simulink model "filterbankFIR"  (R2018a)
settings: Solver=FixedStepDiscrete  StartTime=0.0  StopTime=0.01  RelTol=1e-3
values from neighbouring files (symbols this model uses):
  gainConsts = 10.^(requiredGainDB/10)    [main.m]
  T = table(Band, fm, Lowerfreq, Upperfreq, Fstop2, Fstop1)    [filterbankProto.m]    (also in main.m = 2.26757369615e-05)
undefined symbols (not defined in the file or in its folder): fdesignblkfcn, gcbh
libraries: dspsrcs4 x2, dspfdesign x2, dspxfrm3 x1, dspspect3 x1, dspsigops x1, dspmisc x1, dspmtrx3 x1, dspobslib x1
(part 1 of 5)
settings Model: SimulationMode=accelerator  Creator=Kavi  LastModifiedBy=kavilannair
settings SolverCC: AutoInsertRateTranBlk=on
settings DataIOCC: LimitDataPoints=on  SaveOutput=off  SignalLogging=off  SaveTime=off
settings OptimizationCC: LifeSpan=inf  SimCompilerOptimization=on
settings DebuggingCC: AlgebraicLoopMsg=error  SingleTaskRateTransMsg=error  AllowSymbolicDim=off  SFUnexpectedBacktrackingDiag=warning  SFNoUnconditionalDefaultTransitionDiag=warning  SFExecutionAtInitializationDiag=none
settings CodeAppCC: StateflowObjectComments=on
settings GRTTargetCC: TargetLangStandard=C89/C90 (ANSI)  GeneratePreprocessorConditionals=Disable all
settings ConfigComp: CovMetricSettings=dw  CovHtmlReporting=on  CovSaveCumulativeToWorkspaceVar=on  CovSaveSingleToWorkspaceVar=on  CovExternalEMLEnable=off  CovSFcnEnable=off

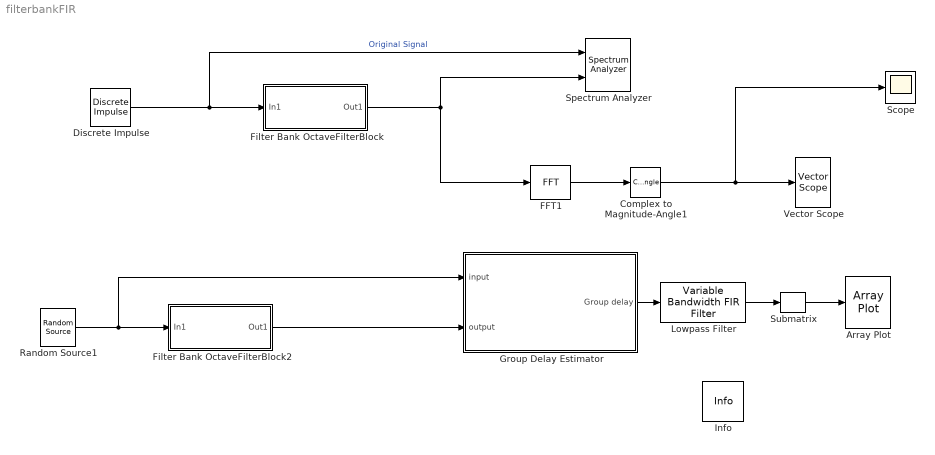
== system filterbankFIR ==
  Array Plot : ArrayPlot
  Complex to Magnitude-Angle1 : ComplexToMagnitudeAngle  Output=Magnitude
  Discrete Impulse : dspsrcs4/Discrete  Impulse  Delay=0  SampleTime=T  FrameSample=512  OutputFrames=off  dataType=double  isSigned=on  wordLen=16  udDataType=sfix(16)  fracBitsMode=Best precision  numFracBits=15  OutDataTypeStr=double  LastOutDataTypeStr=double
  FFT1 : dspxfrm3/FFT  FFTImplementation=Auto  CompMethod=Table lookup  TableOpt=NEW  TableOptActive=Speed  BitRevOrder=off  Normalize=off  InheritFFTLength=on  FFTLength=64  WrapInput=on  roundingMode=Floor  overflowMode=off  firstCoeffDataTypeStr=Inherit: Same word length as input  firstCoeffLastDataTypeStr=Inherit: Same word length as input  outputMin=[]  outputMax=[]
  Filter Bank OctaveFilterBlock : Subsystem
  Filter Bank OctaveFilterBlock2 : Subsystem
  Group Delay Estimator : Subsystem
  Info : dspmisc/Info  SystemSampleTime=-1
      settings: SourceProductName=DSP System Toolbox  SourceProductBaseCode=DS
  Lowpass Filter : dspfdesign/Variable Bandwidth FIR Filter  FilterOrder=30  FilterType=Lowpass  CutoffFrequencyPort=off  CutoffFrequency=fc  CenterFrequencyPort=off  CenterFrequency=1e4  BandwidthPort=off  Bandwidth=2e3  Window=Hann  KaiserWindowParameter=.5  SidelobeAttenuation=60  InheritSampleRate=off  SampleRate=44100  SimulateUsing=Interpreted execution  mask(dsp.simulink.VariableBandwidthFIRFilter){fc=1323.094}
      mask prompts: fc "Cutoff frequency (Hz)"
      mask help: Masked version of dspfdesign/Variable Bandwidth FIR Filter block
      settings: SourceProductName=DSP System Toolbox  SourceProductBaseCode=DS
      mask Display:
      | % This is a new mask on top of the base mask.
      | % Use "View base mask" link below to see the base mask.
      | fprintf('Lowpass filter')
  Random Source1 : dspsrcs4/Random Source  SrcType=Gaussian  NormMethod=Ziggurat  CltLength=12  MinVal=0  MaxVal=1  MeanVal=0  VarVal=1  RepMode=Repeatable  rawSeed=1  IsInherit=off  SampMode=Discrete  SampTime=1/44100  SampFrame=512  DataType=Double  OutComplex=Real  OutputFrames=off
  Scope : Scope
  Spectrum Analyzer : SpectrumAnalyzer  NumInputPorts=2
  Submatrix : dspmtrx3/Submatrix  RowSpan=Range of rows  RowStartMode=Index  RowStartIndex=31  RowEndMode=Last  RowEndIndex=1  ColSpan=All columns  ColStartMode=First  ColStartIndex=1  ColEndMode=Last  ColEndIndex=1
  Vector Scope : dspobslib/Vector Scope  ScopeProperties=off  Domain=Frequency  HorizSpan=1  DisplayProperties=off  AxisGrid=on  Memory=off  FrameNumber=on  AxisLegend=off  AxisZoom=off  OpenScopeAtSimStart=on  OpenScopeImmediately=off  FigPos=[86 244 1118 420]  AxisProperties=on  XUnits=Hertz  XRange=[0...Fs/2]  InheritXIncr=on  XIncr=1  XLabel=Samples  XLimit=Auto  XMin=0  XMax=1  XStart=0  YUnits=dB  YLabel=|Magnitude (dB)|  LineProperties=off  LineMarkers=+  LineColors=[1 0 0]  XAxisParamsVer=6.9
      settings: SourceProductName=DSP System Toolbox  SourceProductBaseCode=DS  YMin=0.0723692553519949  YMax=69.3188381671759
  wires:
  Discrete Impulse/1 -> Spectrum Analyzer/1, Filter Bank OctaveFilterBlock/1(In1)  "Original Signal"
  Complex to Magnitude-Angle1/1 -> Scope/1, Vector Scope/1
  FFT1/1 -> Complex to Magnitude-Angle1/1
  Filter Bank OctaveFilterBlock/1(Out1) -> FFT1/1, Spectrum Analyzer/2
  Filter Bank OctaveFilterBlock2/1(Out1) -> Group Delay Estimator/2(output)
  Group Delay Estimator/1(Group delay) -> Lowpass Filter/1
  Submatrix/1 -> Array Plot/1
  Lowpass Filter/1 -> Submatrix/1
  Random Source1/1 -> Filter Bank OctaveFilterBlock2/1(In1), Group Delay Estimator/1(input)

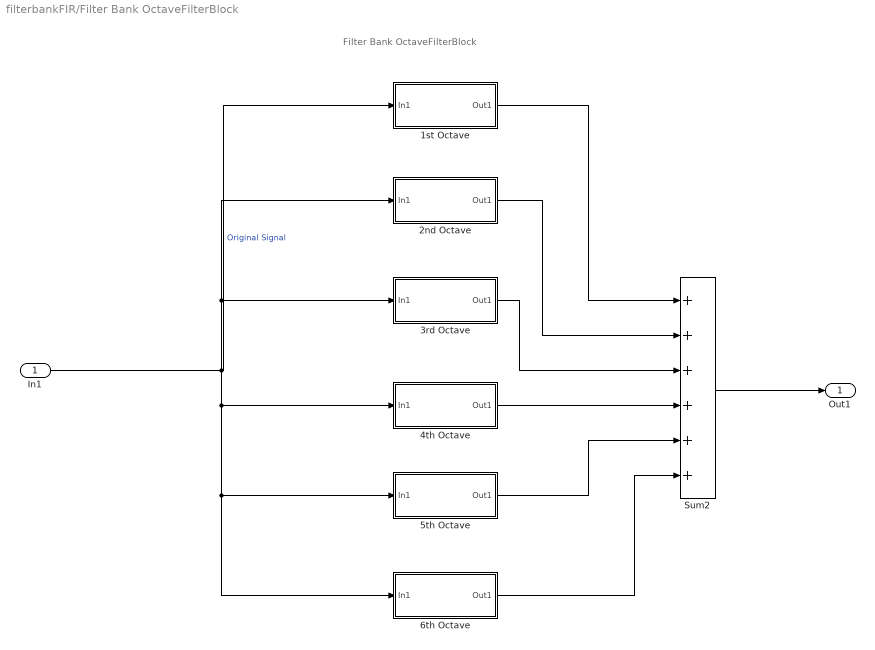
== system filterbankFIR/Filter Bank OctaveFilterBlock ==
  note: Filter Bank OctaveFilterBlock
  In1 : Inport
  "1st Octave " : Subsystem
  2nd Octave : Subsystem
  "3rd Octave " : Subsystem
  4th Octave : Subsystem
  5th Octave : Subsystem
  6th Octave : Subsystem
  Sum2 : Sum  Inputs=++++++
  Out1 : Outport
  wires:
  Sum2/1 -> Out1/1
  "1st Octave "/1(Out1) -> Sum2/1
  2nd Octave/1(Out1) -> Sum2/2
  "3rd Octave "/1(Out1) -> Sum2/3
  4th Octave/1(Out1) -> Sum2/4
  5th Octave/1(Out1) -> Sum2/5
  6th Octave/1(Out1) -> Sum2/6
  In1/1 -> 4th Octave/1(In1), 5th Octave/1(In1), 6th Octave/1(In1), "3rd Octave "/1(In1), 2nd Octave/1(In1), "1st Octave "/1(In1)  "Original Signal"

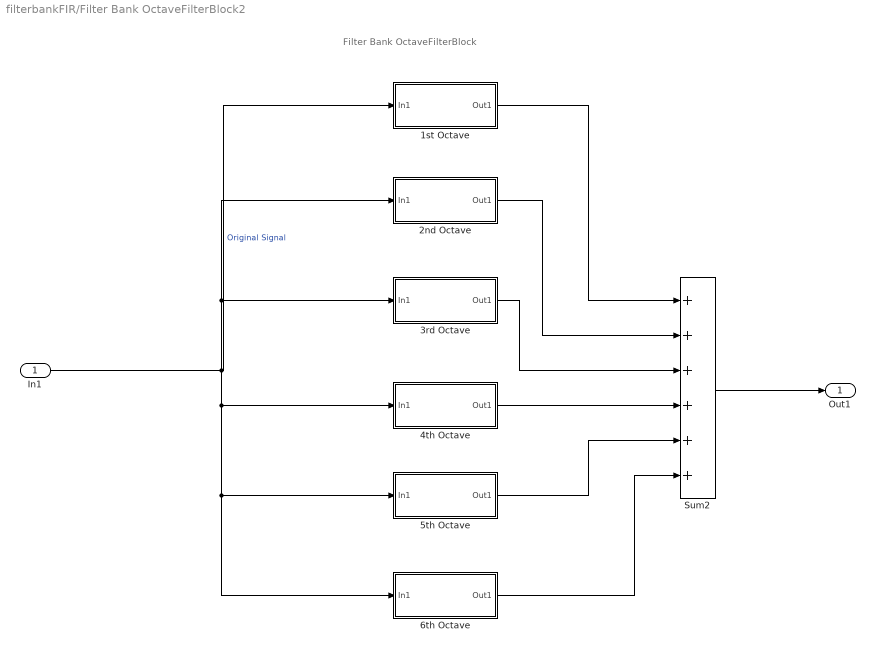
== system filterbankFIR/Filter Bank OctaveFilterBlock2 ==
  note: Filter Bank OctaveFilterBlock
  In1 : Inport
  "1st Octave " : Subsystem
  2nd Octave : Subsystem
  "3rd Octave " : Subsystem
  4th Octave : Subsystem
  5th Octave : Subsystem
  6th Octave : Subsystem
  Sum2 : Sum  Inputs=++++++
  Out1 : Outport
  wires:
  Sum2/1 -> Out1/1
  "1st Octave "/1(Out1) -> Sum2/1
  2nd Octave/1(Out1) -> Sum2/2
  "3rd Octave "/1(Out1) -> Sum2/3
  4th Octave/1(Out1) -> Sum2/4
  5th Octave/1(Out1) -> Sum2/5
  6th Octave/1(Out1) -> Sum2/6
  In1/1 -> 4th Octave/1(In1), 5th Octave/1(In1), 6th Octave/1(In1), "3rd Octave "/1(In1), 2nd Octave/1(In1), "1st Octave "/1(In1)  "Original Signal"

== system filterbankFIR/Group Delay Estimator ==
  input : Inport
  output : Inport  Port=2
  Differentiator Filter : dspfdesign/Differentiator Filter  DesignForMinimumOrder=off  FilterOrder=3  PassbandRipple=0.1  ScaleCoefficients=off  SimulateUsing=Interpreted execution  roundingMode=Floor  coeffsDataTypeStr=fixdt(1,16)
      settings: SourceProductName=DSP System Toolbox  SourceProductBaseCode=DS
  Discrete Transfer Function Estimator : dspspect3/Discrete Transfer Function Estimator  WindowLength=2056  Overlap=0  SpectralAverages=10  FFTLengthSource=Auto  FFTLength=2048  Window=Hann  SidelobeAttenuation=60  FrequencyRange=One-sided  OutputCoherence=off  SimulateUsing=Code generation
      settings: SourceProductName=DSP System Toolbox  SourceProductBaseCode=DS
  Gain1 : Gain  Gain=-22050/257
  Phase Extractor : dspsigops/Phase Extractor  TreatFramesIndependently=on  SimulateUsing=Code generation
      settings: SourceProductName=DSP System Toolbox  SourceProductBaseCode=DS
  Group delay : Outport
  wires:
  output/1 -> Discrete Transfer Function Estimator/2
  Differentiator Filter/1 -> Group delay/1
  input/1 -> Discrete Transfer Function Estimator/1
  Gain1/1 -> Differentiator Filter/1
  Phase Extractor/1 -> Gain1/1
  Discrete Transfer Function Estimator/1 -> Phase Extractor/1

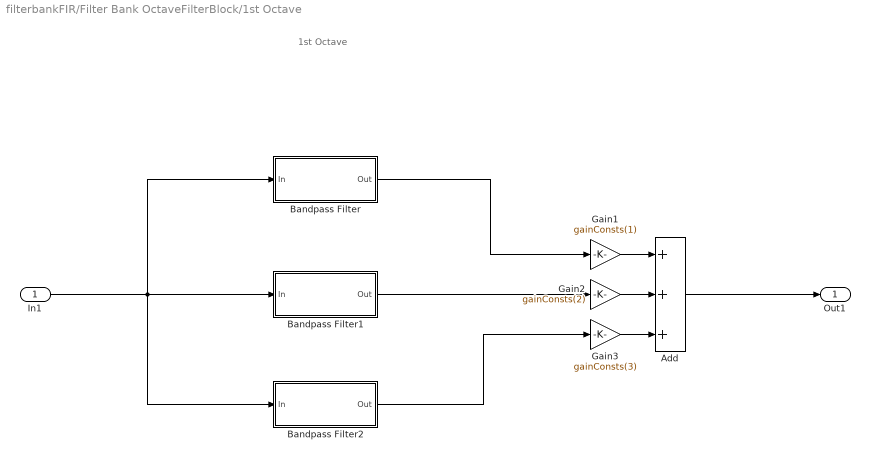
== system filterbankFIR/Filter Bank OctaveFilterBlock/1st Octave  ==
  note: 1st Octave
  In1 : Inport
  Add : Sum  Inputs=+++
  Bandpass Filter : Subsystem  DialogController=fdesignblkfcn  InitFcn=fdesignblkfcn(gcbh, {'InitFcn'});  mask(Bandpass Filter){}
      mask help: Design a bandpass filter
      settings: CopyFcn=fdesignblkfcn(gcbh, {'CopyFcn'});
      mask Help: helpview(mapfilelocation('dsp'), 'dspbandpassfilter');
      mask Display: disp('Bandpass');
  Bandpass Filter1 : Subsystem  DialogController=fdesignblkfcn  InitFcn=fdesignblkfcn(gcbh, {'InitFcn'});  mask(Bandpass Filter){}
      mask help: Design a bandpass filter
      settings: CopyFcn=fdesignblkfcn(gcbh, {'CopyFcn'});
      mask Help: helpview(mapfilelocation('dsp'), 'dspbandpassfilter');
      mask Display: disp('Bandpass');
  Bandpass Filter2 : Subsystem  DialogController=fdesignblkfcn  InitFcn=fdesignblkfcn(gcbh, {'InitFcn'});  mask(Bandpass Filter){}
      mask help: Design a bandpass filter
      settings: CopyFcn=fdesignblkfcn(gcbh, {'CopyFcn'});
      mask Help: helpview(mapfilelocation('dsp'), 'dspbandpassfilter');
      mask Display: disp('Bandpass');
  Gain1 : Gain  Gain=gainConsts(1)
  Gain2 : Gain  Gain=gainConsts(2)
  Gain3 : Gain  Gain=gainConsts(3)
  Out1 : Outport
  wires:
  In1/1 -> Bandpass Filter2/1(In), Bandpass Filter1/1(In), Bandpass Filter/1(In)
  Bandpass Filter1/1(Out) -> Gain2/1
  Bandpass Filter/1(Out) -> Gain1/1
  Bandpass Filter2/1(Out) -> Gain3/1
  Add/1 -> Out1/1
  Gain1/1 -> Add/1
  Gain2/1 -> Add/2
  Gain3/1 -> Add/3

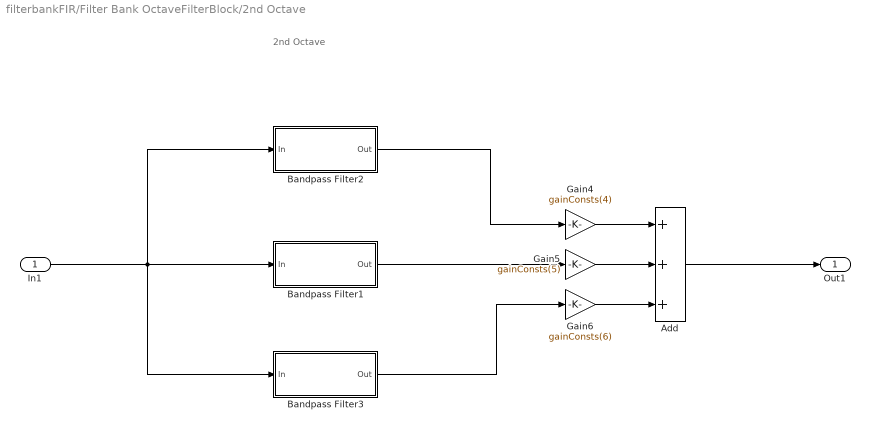
== system filterbankFIR/Filter Bank OctaveFilterBlock/2nd Octave ==
  note: 2nd Octave
  In1 : Inport
  Add : Sum  Inputs=+++
  Bandpass Filter1 : Subsystem  DialogController=fdesignblkfcn  InitFcn=fdesignblkfcn(gcbh, {'InitFcn'});  mask(Bandpass Filter){}
      mask help: Design a bandpass filter
      settings: CopyFcn=fdesignblkfcn(gcbh, {'CopyFcn'});
      mask Help: helpview(mapfilelocation('dsp'), 'dspbandpassfilter');
      mask Display: disp('Bandpass');
  Bandpass Filter2 : Subsystem  DialogController=fdesignblkfcn  InitFcn=fdesignblkfcn(gcbh, {'InitFcn'});  mask(Bandpass Filter){}
      mask help: Design a bandpass filter
      settings: CopyFcn=fdesignblkfcn(gcbh, {'CopyFcn'});
      mask Help: helpview(mapfilelocation('dsp'), 'dspbandpassfilter');
      mask Display: disp('Bandpass');
  Bandpass Filter3 : Subsystem  DialogController=fdesignblkfcn  InitFcn=fdesignblkfcn(gcbh, {'InitFcn'});  mask(Bandpass Filter){}
      mask help: Design a bandpass filter
      settings: CopyFcn=fdesignblkfcn(gcbh, {'CopyFcn'});
      mask Help: helpview(mapfilelocation('dsp'), 'dspbandpassfilter');
      mask Display: disp('Bandpass');
  Gain4 : Gain  Gain=gainConsts(4)
  Gain5 : Gain  Gain=gainConsts(5)
  Gain6 : Gain  Gain=gainConsts(6)
  Out1 : Outport
  wires:
  In1/1 -> Bandpass Filter3/1(In), Bandpass Filter1/1(In), Bandpass Filter2/1(In)
  Bandpass Filter1/1(Out) -> Gain5/1
  Bandpass Filter2/1(Out) -> Gain4/1
  Bandpass Filter3/1(Out) -> Gain6/1
  Add/1 -> Out1/1
  Gain4/1 -> Add/1
  Gain5/1 -> Add/2
  Gain6/1 -> Add/3

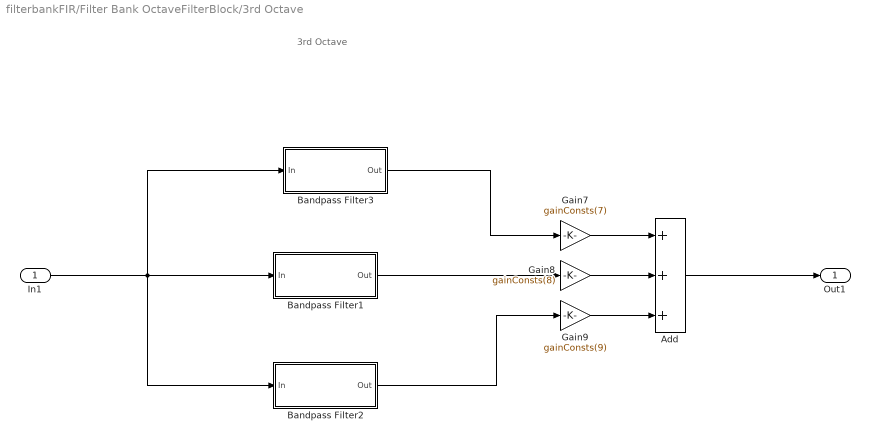
== system filterbankFIR/Filter Bank OctaveFilterBlock/3rd Octave  ==
  note: 3rd Octave
  In1 : Inport
  Add : Sum  Inputs=+++
  Bandpass Filter1 : Subsystem  DialogController=fdesignblkfcn  InitFcn=fdesignblkfcn(gcbh, {'InitFcn'});  mask(Bandpass Filter){}
      mask help: Design a bandpass filter
      settings: CopyFcn=fdesignblkfcn(gcbh, {'CopyFcn'});
      mask Help: helpview(mapfilelocation('dsp'), 'dspbandpassfilter');
      mask Display: disp('Bandpass');
  Bandpass Filter2 : Subsystem  DialogController=fdesignblkfcn  InitFcn=fdesignblkfcn(gcbh, {'InitFcn'});  mask(Bandpass Filter){}
      mask help: Design a bandpass filter
      settings: CopyFcn=fdesignblkfcn(gcbh, {'CopyFcn'});
      mask Help: helpview(mapfilelocation('dsp'), 'dspbandpassfilter');
      mask Display: disp('Bandpass');
  Bandpass Filter3 : Subsystem  DialogController=fdesignblkfcn  InitFcn=fdesignblkfcn(gcbh, {'InitFcn'});  mask(Bandpass Filter){}
      mask help: Design a bandpass filter
      settings: CopyFcn=fdesignblkfcn(gcbh, {'CopyFcn'});
      mask Help: helpview(mapfilelocation('dsp'), 'dspbandpassfilter');
      mask Display: disp('Bandpass');
  Gain7 : Gain  Gain=gainConsts(7)
  Gain8 : Gain  Gain=gainConsts(8)
  Gain9 : Gain  Gain=gainConsts(9)
  Out1 : Outport
  wires:
  In1/1 -> Bandpass Filter2/1(In), Bandpass Filter1/1(In), Bandpass Filter3/1(In)
  Bandpass Filter1/1(Out) -> Gain8/1
  Bandpass Filter3/1(Out) -> Gain7/1
  Bandpass Filter2/1(Out) -> Gain9/1
  Add/1 -> Out1/1
  Gain7/1 -> Add/1
  Gain8/1 -> Add/2
  Gain9/1 -> Add/3

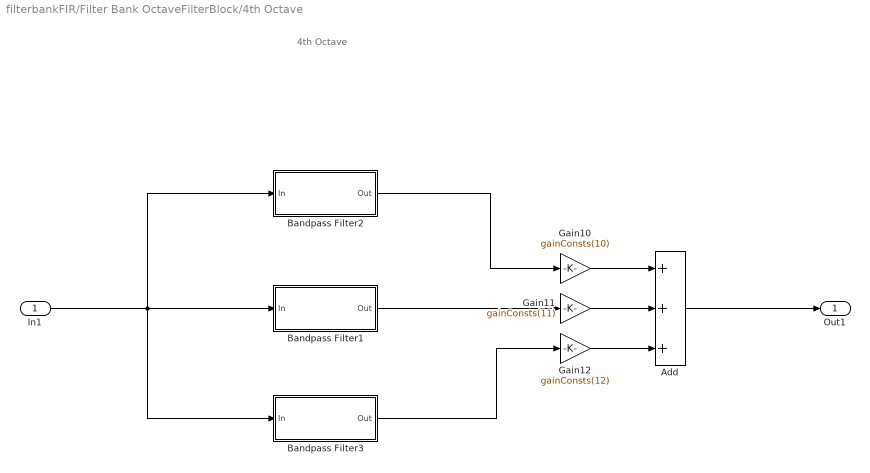
== system filterbankFIR/Filter Bank OctaveFilterBlock/4th Octave ==
  note: 4th Octave
  In1 : Inport
  Add : Sum  Inputs=+++
  Bandpass Filter1 : Subsystem  DialogController=fdesignblkfcn  InitFcn=fdesignblkfcn(gcbh, {'InitFcn'});  mask(Bandpass Filter){}
      mask help: Design a bandpass filter
      settings: CopyFcn=fdesignblkfcn(gcbh, {'CopyFcn'});
      mask Help: helpview(mapfilelocation('dsp'), 'dspbandpassfilter');
      mask Display: disp('Bandpass');
  Bandpass Filter2 : Subsystem  DialogController=fdesignblkfcn  InitFcn=fdesignblkfcn(gcbh, {'InitFcn'});  mask(Bandpass Filter){}
      mask help: Design a bandpass filter
      settings: CopyFcn=fdesignblkfcn(gcbh, {'CopyFcn'});
      mask Help: helpview(mapfilelocation('dsp'), 'dspbandpassfilter');
      mask Display: disp('Bandpass');
  Bandpass Filter3 : Subsystem  DialogController=fdesignblkfcn  InitFcn=fdesignblkfcn(gcbh, {'InitFcn'});  mask(Bandpass Filter){}
      mask help: Design a bandpass filter
      settings: CopyFcn=fdesignblkfcn(gcbh, {'CopyFcn'});
      mask Help: helpview(mapfilelocation('dsp'), 'dspbandpassfilter');
      mask Display: disp('Bandpass');
  Gain10 : Gain  Gain=gainConsts(10)
  Gain11 : Gain  Gain=gainConsts(11)
  Gain12 : Gain  Gain=gainConsts(12)
  Out1 : Outport
  wires:
  In1/1 -> Bandpass Filter3/1(In), Bandpass Filter1/1(In), Bandpass Filter2/1(In)
  Bandpass Filter1/1(Out) -> Gain11/1
  Bandpass Filter2/1(Out) -> Gain10/1
  Bandpass Filter3/1(Out) -> Gain12/1
  Add/1 -> Out1/1
  Gain10/1 -> Add/1
  Gain11/1 -> Add/2
  Gain12/1 -> Add/3

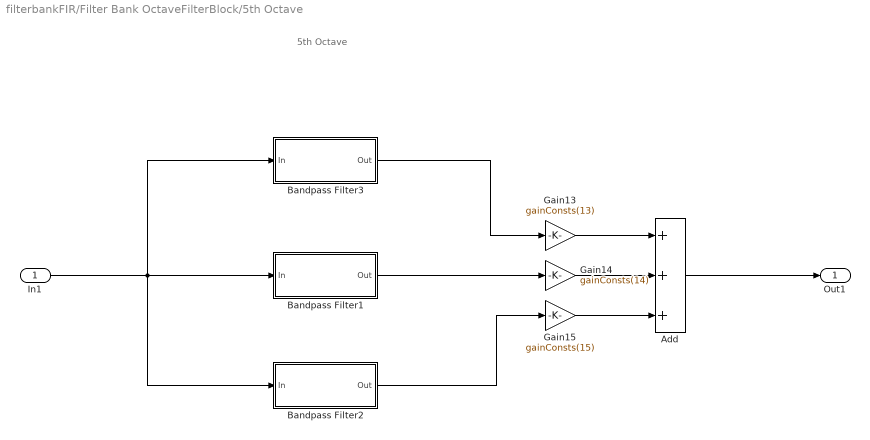
== system filterbankFIR/Filter Bank OctaveFilterBlock/5th Octave ==
  note: 5th Octave
  In1 : Inport
  Add : Sum  Inputs=+++
  Bandpass Filter1 : Subsystem  DialogController=fdesignblkfcn  InitFcn=fdesignblkfcn(gcbh, {'InitFcn'});  mask(Bandpass Filter){}
      mask help: Design a bandpass filter
      settings: CopyFcn=fdesignblkfcn(gcbh, {'CopyFcn'});
      mask Help: helpview(mapfilelocation('dsp'), 'dspbandpassfilter');
      mask Display: disp('Bandpass');
  Bandpass Filter2 : Subsystem  DialogController=fdesignblkfcn  InitFcn=fdesignblkfcn(gcbh, {'InitFcn'});  mask(Bandpass Filter){}
      mask help: Design a bandpass filter
      settings: CopyFcn=fdesignblkfcn(gcbh, {'CopyFcn'});
      mask Help: helpview(mapfilelocation('dsp'), 'dspbandpassfilter');
      mask Display: disp('Bandpass');
  Bandpass Filter3 : Subsystem  DialogController=fdesignblkfcn  InitFcn=fdesignblkfcn(gcbh, {'InitFcn'});  mask(Bandpass Filter){}
      mask help: Design a bandpass filter
      settings: CopyFcn=fdesignblkfcn(gcbh, {'CopyFcn'});
      mask Help: helpview(mapfilelocation('dsp'), 'dspbandpassfilter');
      mask Display: disp('Bandpass');
  "Gain13 " : Gain  Gain=gainConsts(13)
  Gain14 : Gain  Gain=gainConsts(14)
  Gain15 : Gain  Gain=gainConsts(15)
  Out1 : Outport
  wires:
  In1/1 -> Bandpass Filter2/1(In), Bandpass Filter1/1(In), Bandpass Filter3/1(In)
  Bandpass Filter1/1(Out) -> Gain14/1
  Bandpass Filter3/1(Out) -> "Gain13 "/1
  Bandpass Filter2/1(Out) -> Gain15/1
  Add/1 -> Out1/1
  "Gain13 "/1 -> Add/1
  Gain14/1 -> Add/2
  Gain15/1 -> Add/3

== system filterbankFIR/Filter Bank OctaveFilterBlock/6th Octave ==
  note: 6th Octave
  In1 : Inport
  Bandpass Filter2 : Subsystem  DialogController=fdesignblkfcn  InitFcn=fdesignblkfcn(gcbh, {'InitFcn'});  mask(Bandpass Filter){}
      mask help: Design a bandpass filter
      settings: CopyFcn=fdesignblkfcn(gcbh, {'CopyFcn'});
      mask Help: helpview(mapfilelocation('dsp'), 'dspbandpassfilter');
      mask Display: disp('Bandpass');
  Gain16 : Gain  Gain=gainConsts(16)
  Out1 : Outport
  wires:
  In1/1 -> Bandpass Filter2/1(In)
  Bandpass Filter2/1(Out) -> Gain16/1
  Gain16/1 -> Out1/1

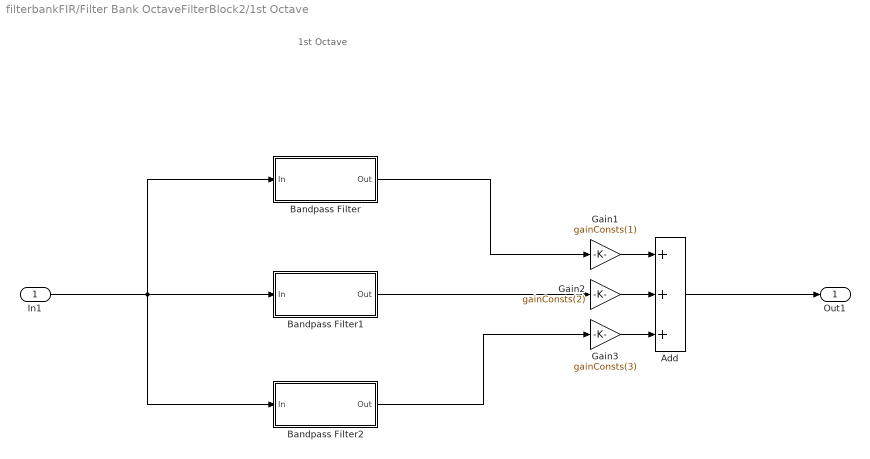
== system filterbankFIR/Filter Bank OctaveFilterBlock2/1st Octave  ==
  note: 1st Octave
  In1 : Inport
  Add : Sum  Inputs=+++
  Bandpass Filter : Subsystem  DialogController=fdesignblkfcn  InitFcn=fdesignblkfcn(gcbh, {'InitFcn'});  mask(Bandpass Filter){}
      mask help: Design a bandpass filter
      settings: CopyFcn=fdesignblkfcn(gcbh, {'CopyFcn'});
      mask Help: helpview(mapfilelocation('dsp'), 'dspbandpassfilter');
      mask Display: disp('Bandpass');
  Bandpass Filter1 : Subsystem  DialogController=fdesignblkfcn  InitFcn=fdesignblkfcn(gcbh, {'InitFcn'});  mask(Bandpass Filter){}
      mask help: Design a bandpass filter
      settings: CopyFcn=fdesignblkfcn(gcbh, {'CopyFcn'});
      mask Help: helpview(mapfilelocation('dsp'), 'dspbandpassfilter');
      mask Display: disp('Bandpass');
  Bandpass Filter2 : Subsystem  DialogController=fdesignblkfcn  InitFcn=fdesignblkfcn(gcbh, {'InitFcn'});  mask(Bandpass Filter){}
      mask help: Design a bandpass filter
      settings: CopyFcn=fdesignblkfcn(gcbh, {'CopyFcn'});
      mask Help: helpview(mapfilelocation('dsp'), 'dspbandpassfilter');
      mask Display: disp('Bandpass');
  Gain1 : Gain  Gain=gainConsts(1)
  Gain2 : Gain  Gain=gainConsts(2)
  Gain3 : Gain  Gain=gainConsts(3)
  Out1 : Outport
  wires:
  In1/1 -> Bandpass Filter2/1(In), Bandpass Filter1/1(In), Bandpass Filter/1(In)
  Bandpass Filter1/1(Out) -> Gain2/1
  Bandpass Filter/1(Out) -> Gain1/1
  Bandpass Filter2/1(Out) -> Gain3/1
  Add/1 -> Out1/1
  Gain1/1 -> Add/1
  Gain2/1 -> Add/2
  Gain3/1 -> Add/3

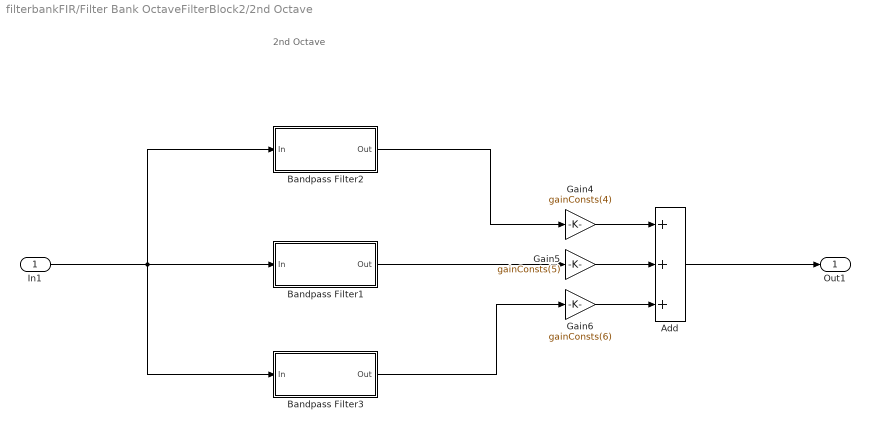
== system filterbankFIR/Filter Bank OctaveFilterBlock2/2nd Octave ==
  note: 2nd Octave
  In1 : Inport
  Add : Sum  Inputs=+++
  Bandpass Filter1 : Subsystem  DialogController=fdesignblkfcn  InitFcn=fdesignblkfcn(gcbh, {'InitFcn'});  mask(Bandpass Filter){}
      mask help: Design a bandpass filter
      settings: CopyFcn=fdesignblkfcn(gcbh, {'CopyFcn'});
      mask Help: helpview(mapfilelocation('dsp'), 'dspbandpassfilter');
      mask Display: disp('Bandpass');
  Bandpass Filter2 : Subsystem  DialogController=fdesignblkfcn  InitFcn=fdesignblkfcn(gcbh, {'InitFcn'});  mask(Bandpass Filter){}
      mask help: Design a bandpass filter
      settings: CopyFcn=fdesignblkfcn(gcbh, {'CopyFcn'});
      mask Help: helpview(mapfilelocation('dsp'), 'dspbandpassfilter');
      mask Display: disp('Bandpass');
  Bandpass Filter3 : Subsystem  DialogController=fdesignblkfcn  InitFcn=fdesignblkfcn(gcbh, {'InitFcn'});  mask(Bandpass Filter){}
      mask help: Design a bandpass filter
      settings: CopyFcn=fdesignblkfcn(gcbh, {'CopyFcn'});
      mask Help: helpview(mapfilelocation('dsp'), 'dspbandpassfilter');
      mask Display: disp('Bandpass');
  Gain4 : Gain  Gain=gainConsts(4)
  Gain5 : Gain  Gain=gainConsts(5)
  Gain6 : Gain  Gain=gainConsts(6)
  Out1 : Outport
  wires:
  In1/1 -> Bandpass Filter3/1(In), Bandpass Filter1/1(In), Bandpass Filter2/1(In)
  Bandpass Filter1/1(Out) -> Gain5/1
  Bandpass Filter2/1(Out) -> Gain4/1
  Bandpass Filter3/1(Out) -> Gain6/1
  Add/1 -> Out1/1
  Gain4/1 -> Add/1
  Gain5/1 -> Add/2
  Gain6/1 -> Add/3

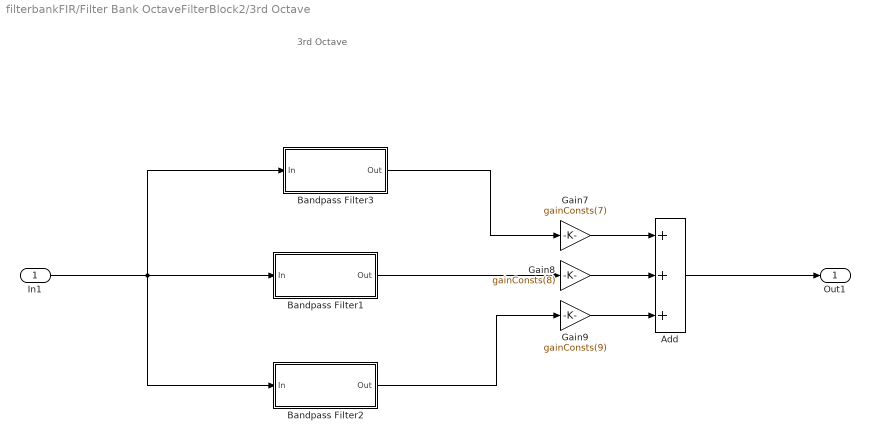
== system filterbankFIR/Filter Bank OctaveFilterBlock2/3rd Octave  ==
  note: 3rd Octave
  In1 : Inport
  Add : Sum  Inputs=+++
  Bandpass Filter1 : Subsystem  DialogController=fdesignblkfcn  InitFcn=fdesignblkfcn(gcbh, {'InitFcn'});  mask(Bandpass Filter){}
      mask help: Design a bandpass filter
      settings: CopyFcn=fdesignblkfcn(gcbh, {'CopyFcn'});
      mask Help: helpview(mapfilelocation('dsp'), 'dspbandpassfilter');
      mask Display: disp('Bandpass');
  Bandpass Filter2 : Subsystem  DialogController=fdesignblkfcn  InitFcn=fdesignblkfcn(gcbh, {'InitFcn'});  mask(Bandpass Filter){}
      mask help: Design a bandpass filter
      settings: CopyFcn=fdesignblkfcn(gcbh, {'CopyFcn'});
      mask Help: helpview(mapfilelocation('dsp'), 'dspbandpassfilter');
      mask Display: disp('Bandpass');
  Bandpass Filter3 : Subsystem  DialogController=fdesignblkfcn  InitFcn=fdesignblkfcn(gcbh, {'InitFcn'});  mask(Bandpass Filter){}
      mask help: Design a bandpass filter
      settings: CopyFcn=fdesignblkfcn(gcbh, {'CopyFcn'});
      mask Help: helpview(mapfilelocation('dsp'), 'dspbandpassfilter');
      mask Display: disp('Bandpass');
  Gain7 : Gain  Gain=gainConsts(7)
  Gain8 : Gain  Gain=gainConsts(8)
  Gain9 : Gain  Gain=gainConsts(9)
  Out1 : Outport
  wires:
  In1/1 -> Bandpass Filter2/1(In), Bandpass Filter1/1(In), Bandpass Filter3/1(In)
  Bandpass Filter1/1(Out) -> Gain8/1
  Bandpass Filter3/1(Out) -> Gain7/1
  Bandpass Filter2/1(Out) -> Gain9/1
  Add/1 -> Out1/1
  Gain7/1 -> Add/1
  Gain8/1 -> Add/2
  Gain9/1 -> Add/3

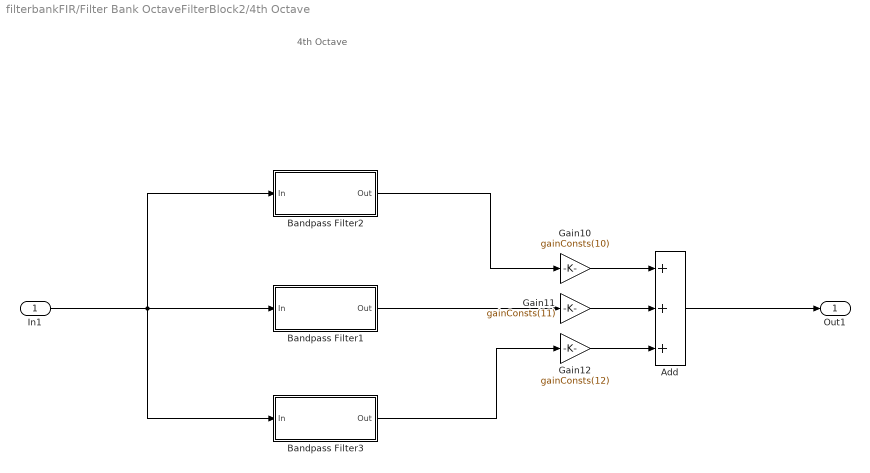
== system filterbankFIR/Filter Bank OctaveFilterBlock2/4th Octave ==
  note: 4th Octave
  In1 : Inport
  Add : Sum  Inputs=+++
  Bandpass Filter1 : Subsystem  DialogController=fdesignblkfcn  InitFcn=fdesignblkfcn(gcbh, {'InitFcn'});  mask(Bandpass Filter){}
      mask help: Design a bandpass filter
      settings: CopyFcn=fdesignblkfcn(gcbh, {'CopyFcn'});
      mask Help: helpview(mapfilelocation('dsp'), 'dspbandpassfilter');
      mask Display: disp('Bandpass');
  Bandpass Filter2 : Subsystem  DialogController=fdesignblkfcn  InitFcn=fdesignblkfcn(gcbh, {'InitFcn'});  mask(Bandpass Filter){}
      mask help: Design a bandpass filter
      settings: CopyFcn=fdesignblkfcn(gcbh, {'CopyFcn'});
      mask Help: helpview(mapfilelocation('dsp'), 'dspbandpassfilter');
      mask Display: disp('Bandpass');
  Bandpass Filter3 : Subsystem  DialogController=fdesignblkfcn  InitFcn=fdesignblkfcn(gcbh, {'InitFcn'});  mask(Bandpass Filter){}
      mask help: Design a bandpass filter
      settings: CopyFcn=fdesignblkfcn(gcbh, {'CopyFcn'});
      mask Help: helpview(mapfilelocation('dsp'), 'dspbandpassfilter');
      mask Display: disp('Bandpass');
  Gain10 : Gain  Gain=gainConsts(10)
  Gain11 : Gain  Gain=gainConsts(11)
  Gain12 : Gain  Gain=gainConsts(12)
  Out1 : Outport
  wires:
  In1/1 -> Bandpass Filter3/1(In), Bandpass Filter1/1(In), Bandpass Filter2/1(In)
  Bandpass Filter1/1(Out) -> Gain11/1
  Bandpass Filter2/1(Out) -> Gain10/1
  Bandpass Filter3/1(Out) -> Gain12/1
  Add/1 -> Out1/1
  Gain10/1 -> Add/1
  Gain11/1 -> Add/2
  Gain12/1 -> Add/3

== system filterbankFIR/Filter Bank OctaveFilterBlock2/5th Octave ==
  note: 5th Octave
  In1 : Inport
  Add : Sum  Inputs=+++
  Bandpass Filter1 : Subsystem  DialogController=fdesignblkfcn  InitFcn=fdesignblkfcn(gcbh, {'InitFcn'});  mask(Bandpass Filter){}
      mask help: Design a bandpass filter
      settings: CopyFcn=fdesignblkfcn(gcbh, {'CopyFcn'});
      mask Help: helpview(mapfilelocation('dsp'), 'dspbandpassfilter');
      mask Display: disp('Bandpass');
  Bandpass Filter2 : Subsystem  DialogController=fdesignblkfcn  InitFcn=fdesignblkfcn(gcbh, {'InitFcn'});  mask(Bandpass Filter){}
      mask help: Design a bandpass filter
      settings: CopyFcn=fdesignblkfcn(gcbh, {'CopyFcn'});
      mask Help: helpview(mapfilelocation('dsp'), 'dspbandpassfilter');
      mask Display: disp('Bandpass');
  Bandpass Filter3 : Subsystem  DialogController=fdesignblkfcn  InitFcn=fdesignblkfcn(gcbh, {'InitFcn'});  mask(Bandpass Filter){}
      mask help: Design a bandpass filter
      settings: CopyFcn=fdesignblkfcn(gcbh, {'CopyFcn'});
      mask Help: helpview(mapfilelocation('dsp'), 'dspbandpassfilter');
      mask Display: disp('Bandpass');
  "Gain13 " : Gain  Gain=gainConsts(13)
  Gain14 : Gain  Gain=gainConsts(14)
  Gain15 : Gain  Gain=gainConsts(15)
  Out1 : Outport
  wires:
  In1/1 -> Bandpass Filter2/1(In), Bandpass Filter1/1(In), Bandpass Filter3/1(In)
  Bandpass Filter1/1(Out) -> Gain14/1
  Bandpass Filter3/1(Out) -> "Gain13 "/1
  Bandpass Filter2/1(Out) -> Gain15/1
  Add/1 -> Out1/1
  "Gain13 "/1 -> Add/1
  Gain14/1 -> Add/2
  Gain15/1 -> Add/3

== system filterbankFIR/Filter Bank OctaveFilterBlock2/6th Octave ==
  note: 6th Octave
  In1 : Inport
  Bandpass Filter2 : Subsystem  DialogController=fdesignblkfcn  InitFcn=fdesignblkfcn(gcbh, {'InitFcn'});  mask(Bandpass Filter){}
      mask help: Design a bandpass filter
      settings: CopyFcn=fdesignblkfcn(gcbh, {'CopyFcn'});
      mask Help: helpview(mapfilelocation('dsp'), 'dspbandpassfilter');
      mask Display: disp('Bandpass');
  Gain16 : Gain  Gain=gainConsts(16)
  Out1 : Outport
  wires:
  In1/1 -> Bandpass Filter2/1(In)
  Bandpass Filter2/1(Out) -> Gain16/1
  Gain16/1 -> Out1/1

== system filterbankFIR/Filter Bank OctaveFilterBlock/1st Octave /Bandpass Filter ==
  In : Inport
  Generated Filter Block : DiscreteFir  Tag=BlockMethodSubSystem  Coefficients=[0.000697642726900061898 8.09552427272728785e-05 8.54298578400442639e-05 8.98807771459664761e-05 9.43384731455670006e-05 9.87461148585240788e-05 0.00010312821470486701 0.000107425015934631512 0.000111661748195207504 0.000115768831845649133 0.00011977430759990099 0.000123604129136607282 0.000127288473311339698 0.000130754241930446531 0.000134037240931339594 0.000137069071879046875 0.000139898927035997888 0.000142458720440894723 0.000144810280725432013 0.000146872586783241584 0.000148709930700294734 0.000150201978029776043 0.000151403116753598313 0.000152140165834634372 0.000152474603526873108 0.000152217746894057191 0.000151532783028162179 0.000150310825384055336 0.000148956765929328941 0.000147305978377082096 0.000145601480761968461 0.000141258575406091923 0.000138350565419553492 0.000134320704794821817 0.000129544803269516216 0.000124378433418626775 0.000118463217933620471 0.000112044630974412123 0.00010491070451036004 9.72232987136207612e-05 8.88346993527331378e-05 7.98625720519617241e-05 7.01890483858774055e-05 5.99025227476447419e-05 4.89011331907505207e-05 3.72578170326489874e-05 2.48912133468461839e-05 1.18703403813766488e-05 -1.85610690242223592e-06 -1.62180853669531029e-05 -3.12436403993010108e-05 -4.68839464801328124e-05 -6.31674983141896626e-05 -8.00879427766511341e-05 -9.76716364688186961e-05 -0.000115914138067600391 -0.000134771279906796147 -0.000154182692472707643 -0.000174049820877978181 -0.000194454480910275434 -0.000215442225699886286 -0.000237219536085798657 -0.000258893442529644063 -0.000281328181419072867 -0.000304168718070202968 -0.000327239169396420233 -0.000350773168512199228 -0.000374506139266087413 -0.000398583831707912111 -0.000422809926581896452 -0.000447270802584624674 -0.000471798209508104928 -0.000496451690074088659 -0.000521081775668509302 -0.000545738210587069089 -0.000570284710026425245 -0.00059476301862592426 -0.000619040766477897599 -0.000643137935610667072 -0.000666917334577428098 -0.000690379819871509088 -0.000713401502760758056 -0.000735984267607486808 -0.000758034203473897114 -0.000779545749287828375 -0.000800415971256329662 -0.000820593423482372103 -0.000839959337644514492 -0.000858487199118198718 -0.000876154221470121729 -0.000892930780525496345 -0.000908697251959440701 -0.000923208719255517139 -0.000936774076257655165 -0.000949083050326562667 -0.000960045589669965282 -0.000969794071301856189 -0.000978060592401867792 -0.000984968388757884519 -0.000990312937434469596 -0.000994163806694911122 -0.000996349911771248018 -0.000996920001307780588 -0.000995722447944197677 -0.000992802724610341658 -0.000988026641477879634 -0.00098144298996558142 -0.000972926889726441219 -0.000962518336166140486 -0.0009500967468750864 -0.00093569801619023112 -0.000919221712658873876 -0.000900712804478870149 -0.000880096230077544823 -0.000857407499502278758 -0.000832565395515348725 -0.000805588167496494633 -0.000776413943030325048 -0.000745109403174732299 -0.000711650884194117749 -0.000676059073999672614 -0.000638264114795646553 -0.000598302643212084281 -0.000556301289770442923 -0.000512126006163914549 -0.000465822496930438923 -0.000417538569238844225 -0.000367124764988179875 -0.000314793686684752036 -0.0002604390314748916 -0.00020422949628435763 -0.000146104031239268641 -8.62146709836672401e-05 -2.45239000581840289e-05 3.88143474971966516e-05 0.000103817183184339062 0.00017032366955133308 0.000238341893868718044 0.000307713180237506058 0.000378435901314149717 0.000450345888544420928 0.000523418511227943003 0.000597479128465274486 0.000672486077885831274 0.000748277634060490193 0.000824813392825104455 0.000901931408300662616 0.000979563007715600863 0.00105751403430597501 0.00113572333046903749 0.00121403139995550986 0.00129236628995358684 0.00137051886224509177 0.00144837230964598774 0.00152584781380884463 0.00160277773696920517 0.00167895613970400672 0.00175438461274487882 0.0018287565877008298 0.00190207603411469799 0.00197407501525775648 0.00204471603430592249 0.00211376017781161971 0.00218115246479933878 ...(+12798 chars)]  InputProcessing=Columns as channels (frame based)
  Out : Outport
  wires:
  In/1 -> Generated Filter Block/1
  Generated Filter Block/1 -> Out/1
